simulink model "a4_fig4"  (R2021b)
settings: Solver=VariableStepAuto  StartTime=0.0  StopTime=10.0  RelTol=1e-3
undefined symbols (not defined in the file or in its folder): denG1, denG2, denG3, denG4, denG5, denH1, dentol0, numG1, numG2, numG3, numG4, numG5, numH1, numtol0
libraries: cstblocks x1
settings Model: Creator=andre  LastModifiedBy=andre

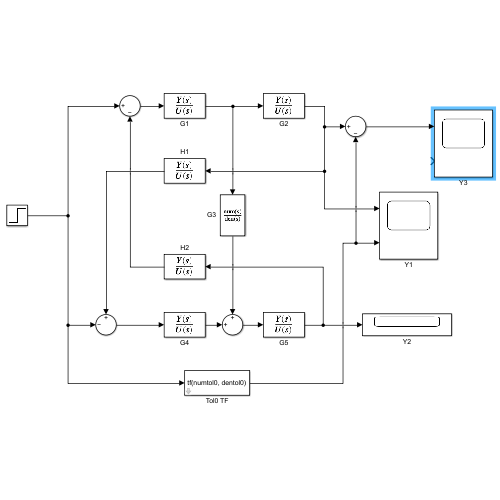
[thumbnail: Simulink's stored preview of the top-level diagram]
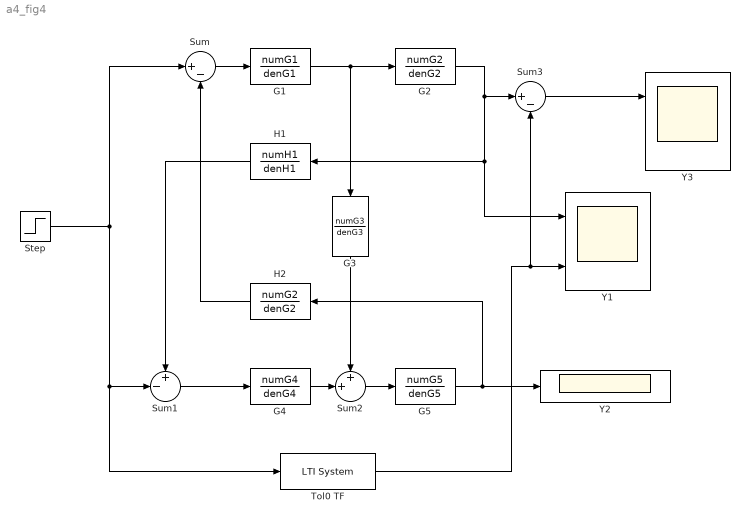
== system a4_fig4 ==
  G1 : TransferFcn  Numerator=numG1  Denominator=denG1
  G2 : TransferFcn  Numerator=numG2  Denominator=denG2
  G3 : TransferFcn  Numerator=numG3  Denominator=denG3
  G4 : TransferFcn  Numerator=numG4  Denominator=denG4
  G5 : TransferFcn  Numerator=numG5  Denominator=denG5
  H1 : TransferFcn  Numerator=numH1  Denominator=denH1
  H2 : TransferFcn  Numerator=numG2  Denominator=denG2
  Step : Step  SampleTime=0
  Sum : Sum  Inputs=|+-
  Sum1 : Sum  Inputs=+-|
  Sum2 : Sum  Inputs=++|
  Sum3 : Sum  Inputs=|+-
  Tol0 TF : cstblocks/LTI System  sys=tf(numtol0, dentol0)  IC=[]
  Y1 : Scope  NumInputPorts=2
  Y2 : Scope
  Y3 : Scope  NumInputPorts=2
  wires:
  Step/1 -> Tol0 TF/1, Sum1/2, Sum/1
  Sum/1 -> G1/1
  G1/1 -> G2/1, G3/1
  G2/1 -> Y1/1, H1/1, Sum3/1
  H1/1 -> Sum1/1
  G4/1 -> Sum2/2
  G3/1 -> Sum2/1
  H2/1 -> Sum/2
  Sum2/1 -> G5/1
  G5/1 -> H2/1, Y2/1
  Tol0 TF/1 -> Y1/2, Sum3/2
  Sum1/1 -> G4/1
  Sum3/1 -> Y3/1
